simulink model "baseon_xr_iter1"  (R2017a)
settings: Solver=VariableStepAuto  StartTime=0.0  StopTime=10  RelTol=1e-3
PreLoadFcn:
  | init.m;
libraries: simulink x1
settings Model: Creator=Administrator  LastModifiedBy=Administrator
settings SolverCC: ZeroCrossAlgorithm=Adaptive  AlgebraicLoopSolver=LineSearch
settings DebuggingCC: MaxConsecutiveZCsMsg=none

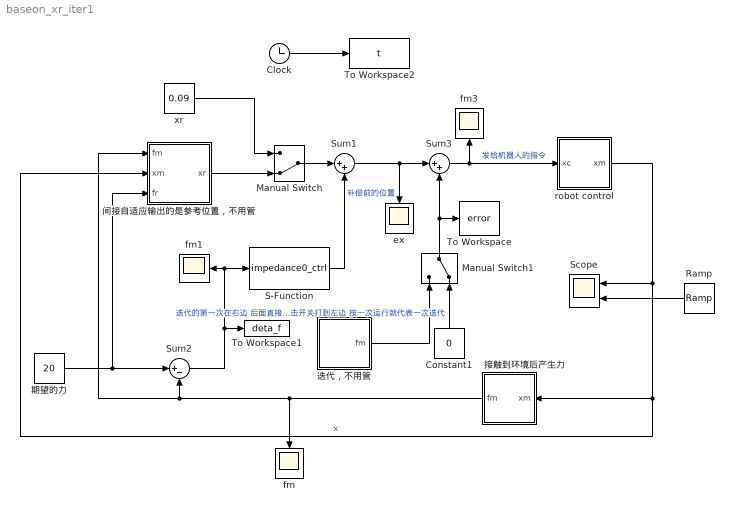
== system baseon_xr_iter1 ==
  Clock : Clock
  Constant1 : Constant  Value=0
  Manual Switch : ManualSwitch  CurrentSetting=0
  Manual Switch1 : ManualSwitch  CurrentSetting=0
  Ramp : simulink/Sources/Ramp  slope=1  start=0  X0=0
  S-Function : S-Function  FunctionName=impedance0_ctrl  SFunctionDeploymentMode=off  EnableBusSupport=off
  Scope : Scope  NumInputPorts=2
  Sum1 : Sum  Inputs=|++
  Sum2 : Sum  Inputs=|+-
  Sum3 : Sum  Inputs=|++
  To Workspace : ToWorkspace  VariableName=error  SampleTime=-1
      settings: Save2DSignal=2-D array (concatenate along first dimension)
  To Workspace1 : ToWorkspace  VariableName=deta_f  SampleTime=-1
      settings: Save2DSignal=2-D array (concatenate along first dimension)
  To Workspace2 : ToWorkspace  VariableName=t  SampleTime=-1
  ex : Scope
  fm : Scope
  fm1 : Scope
  fm3 : Scope
  robot control : Subsystem
  xr : Constant  Value=0.09
  接触到环境后产生力 : Subsystem
  期望的力 : Constant  Value=20
  迭代，不用管 : Subsystem
  间接自适应输出的是参考位置，不用管 : Subsystem
  wires:
  间接自适应输出的是参考位置，不用管/1(xr) -> Manual Switch/2
  xr/1 -> Manual Switch/1
  Manual Switch/1 -> Sum1/1
  期望的力/1 -> 间接自适应输出的是参考位置，不用管/3(fr), Sum2/1
  Sum1/1 -> ex/1, Sum3/1  "补偿前的位置"
  Manual Switch1/1 -> To Workspace/1, Sum3/2
  Constant1/1 -> Manual Switch1/2  "迭代的第一次在右边 后面直接双击开关打到左边 按一次运行就代表一次迭代"
  Sum3/1 -> robot control/1(xc), fm3/1  "发给机器人的指令"
  robot control/1("xm ") -> 间接自适应输出的是参考位置，不用管/2(xm), 接触到环境后产生力/1(xm), Scope/1  "x"
  接触到环境后产生力/1("fm ") -> 间接自适应输出的是参考位置，不用管/1(fm), Sum2/2, fm/1
  Ramp/1 -> Scope/2
  S-Function/1 -> Sum1/2
  Sum2/1 -> fm1/1, S-Function/1, To Workspace1/1
  迭代，不用管/1("fm ") -> Manual Switch1/1
  Clock/1 -> To Workspace2/1

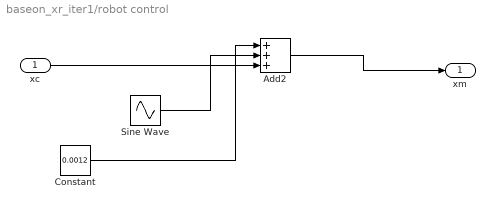
== system baseon_xr_iter1/robot control ==
  xc : Inport
  Add2 : Sum  Inputs=+++
  Constant : Constant  Value=0.0012
  Sine Wave : Sin  Amplitude=0.001  Frequency=0.22  SampleTime=0.01
  "xm " : Outport
  wires:
  xc/1 -> Add2/3
  Add2/1 -> "xm "/1
  Sine Wave/1 -> Add2/2
  Constant/1 -> Add2/1

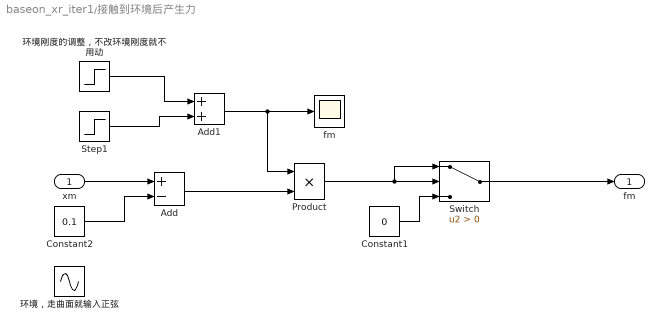
== system baseon_xr_iter1/接触到环境后产生力 ==
  xm : Inport
  Add : Sum  Inputs=+-
  Add1 : Sum
  Constant1 : Constant  Value=0
  Constant2 : Constant  Value=0.1
  Product : Product
  Step1 : Step  Time=1000  After=1500  SampleTime=0
  Switch : Switch  Criteria=u2 > Threshold
  fm : Scope
  环境刚度的调整，不改环境刚度就不用动 : Step  Time=100  Before=1500  After=2500  SampleTime=0
  环境，走曲面就输入正弦 : Sin  Amplitude=0.01  SampleTime=0
  "fm " : Outport
  wires:
  Add1/1 -> Product/1, fm/1
  xm/1 -> Add/1
  Add/1 -> Product/2
  Product/1 -> Switch/1, Switch/2
  Constant1/1 -> Switch/3
  环境刚度的调整，不改环境刚度就不用动/1 -> Add1/1
  Step1/1 -> Add1/2
  Switch/1 -> "fm "/1
  Constant2/1 -> Add/2

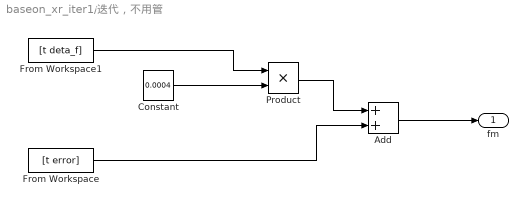
== system baseon_xr_iter1/迭代，不用管 ==
  Add : Sum
  Constant : Constant  Value=0.0004
  From Workspace : FromWorkspace  VariableName=[t error]  SampleTime=0
  From Workspace1 : FromWorkspace  VariableName=[t deta_f]  SampleTime=0
  Product : Product
  "fm " : Outport
  wires:
  Constant/1 -> Product/2
  Product/1 -> Add/1
  From Workspace/1 -> Add/2
  Add/1 -> "fm "/1
  From Workspace1/1 -> Product/1

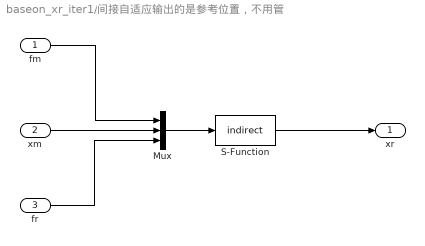
== system baseon_xr_iter1/间接自适应输出的是参考位置，不用管 ==
  fm : Inport
  xm : Inport  Port=2
  fr : Inport  Port=3
  Mux : Mux  Inputs=3
  S-Function : S-Function  FunctionName=indirect  SFunctionDeploymentMode=off  EnableBusSupport=off
  xr : Outport
  wires:
  fm/1 -> Mux/1
  xm/1 -> Mux/2
  Mux/1 -> S-Function/1
  S-Function/1 -> xr/1
  fr/1 -> Mux/3
